simulink model "RLC_circuit"  (R2020b)
settings: Solver=VariableStepAuto  StartTime=0.0  StopTime=0.04  RelTol=1e-3
settings Model: Creator=kjartan  LastModifiedBy=kjartan

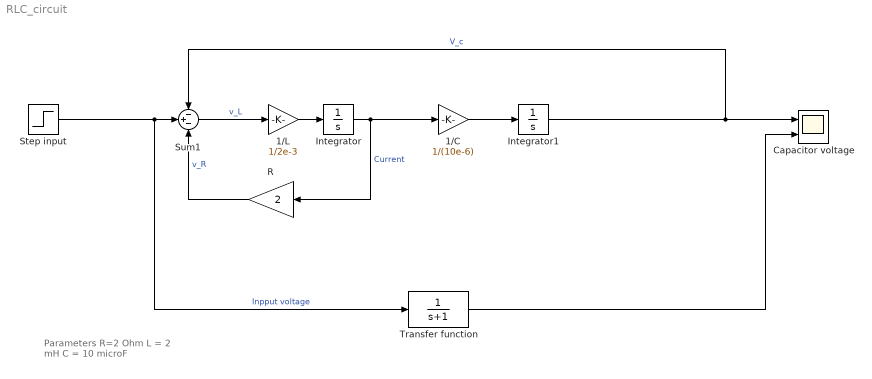
== system RLC_circuit ==
  note: Parameters
      |
      | R=2 Ohm
      | L = 2 mH
      | C = 10 microF
  1/C : Gain  Gain=1/(10e-6)
  1/L : Gain  Gain=1/2e-3
  Capacitor voltage : Scope  NumInputPorts=2
  Integrator : Integrator
  Integrator1 : Integrator
  R : Gain  Gain=2
  Step input : Step  Time=0.01  After=20  SampleTime=0
  Sum1 : Sum  Inputs=-+-
  Transfer function : TransferFcn  Denominator=[1 1]
  wires:
  Integrator1/1 -> Sum1/1, Capacitor voltage/1  "V_c"
  Integrator/1 -> R/1, 1/C/1  "Current"
  1/L/1 -> Integrator/1
  R/1 -> Sum1/3  "v_R"
  Sum1/1 -> 1/L/1  "v_L"
  Step input/1 -> Transfer function/1, Sum1/2  "Inpput voltage"
  Transfer function/1 -> Capacitor voltage/2
  1/C/1 -> Integrator1/1
